simulink model "wwtp"  (R2022a)
settings: Solver=ode23t  StartTime=0.0  StopTime=inf  FixedStep=1E-4  MaxStep=100  RelTol=1e-4  EnableMultiTasking=on
InitFcn:
  | iniASU_UNIT
model workspace (MAT data in the model file):
  Port = 10001
  Port2 = 50001
  RemoteIP = '0.0.0.0'
values from neighbouring files (symbols this model uses):
  Arrhenius = ones(1,15)    [iniASM1model.m]
  Esteq = zeros(NUMREACCIONESBIOL,NUMESTADOSMODASM1)    [iniASM1model.m]
undefined symbols (not defined in the file or in its folder): Cineticos20, Param_ASU_D, Param_ASU_N, Param_Settler_Fns, ParamsEsteq, VarManip_D, VarManip_N, VarManip_QRF, x0_D, x0_N
libraries: dspnetwork x7
settings Model: PacingRate=0.890000  Creator=iirizar  LastModifiedBy=operezdearriluzea
settings SolverCC: InitialStep=1E-22  MaxConsecutiveMinStep=auto  AlgebraicLoopSolver=TrustRegion  SolverResetMethod=Robust
settings DataIOCC: LimitDataPoints=on  MaxDataPoints=1  SaveFinalState=on  SaveFormat=Array  SignalLoggingSaveFormat=ModelDataLogs  SaveOutput=off  SaveState=on  SignalLogging=off  SaveTime=off  ReturnWorkspaceOutputs=off
settings OptimizationCC: ExpressionDepthLimit=2147483647  LifeSpan=inf
settings DebuggingCC: UnderspecifiedInitializationDetection=Classic  MergeDetectMultiDrivingBlocksExec=none  SolverPrmCheckMsg=warning  FcnCallInpInsideContextMsg=warning  UnconnectedInputMsg=warning  UnconnectedOutputMsg=warning  UnconnectedLineMsg=warning  StateNameClashWarn=warning  SFUnexpectedBacktrackingDiag=warning  SFNoUnconditionalDefaultTransitionDiag=warning  SFExecutionAtInitializationDiag=none  SFMachineParentedDataDiag=warning  ArithmeticOperatorsInVariantConditions=warning
settings HardwareCC: ProdBitPerPointer=32  ProdBitPerSizeT=32  ProdBitPerPtrDiffT=32  ProdLargestAtomicFloat=None  ProdIntDivRoundTo=Undefined  ProdEndianess=Unspecified  ProdWordSize=32  ProdHWDeviceType=32-bit Generic
settings ModelReferenceCC: PropagateSignalLabelsOutOfModel=off
settings SFSimCC: SimUseLocalCustomCode=off  CustomCodeUndefinedFunction=UseInterfaceOnly
settings RTWCC: RTWUseLocalCustomCode=off  DLArmComputeVersion=19.05
settings CodeAppCC: StateflowObjectComments=on
settings GRTTargetCC: TargetLangStandard=C89/C90 (ANSI)  CombineOutputUpdateFcns=off  GRTInterface=on
settings ConfigComp: CovMetricSettings=dw  CovSaveCumulativeToWorkspaceVar=on  CovSaveSingleToWorkspaceVar=on  CovExternalEMLEnable=off

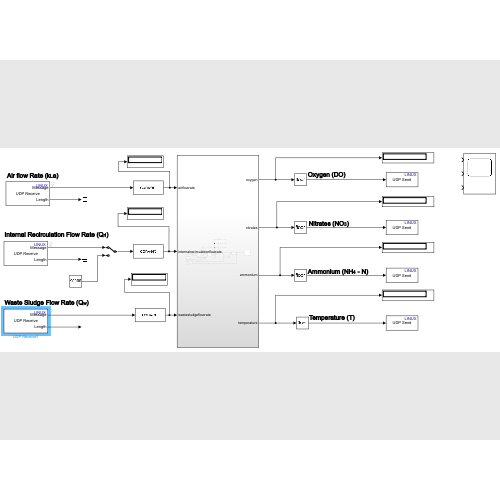
[thumbnail: Simulink's stored preview of the top-level diagram]
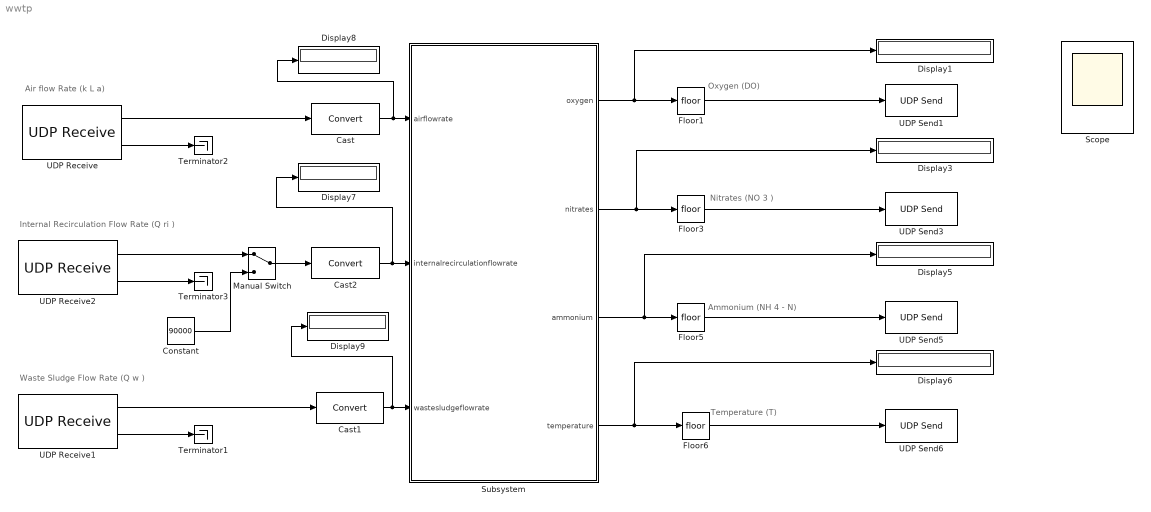
== system wwtp ==
  note: Air flow Rate (k L a)
  note: Waste Sludge Flow Rate (Q w )
  note: Internal Recirculation Flow Rate (Q ri )
  note: Oxygen (DO)
  note: Nitrates (NO 3 )
  note: Ammonium (NH 4 - N)
  note: Temperature (T)
  Cast : DataTypeConversion  OutMin=[0]  OutMax=[1000]  SaturateOnIntegerOverflow=off  RndMeth=Floor
  Cast1 : DataTypeConversion  OutMin=[0]  OutMax=[10000]  SaturateOnIntegerOverflow=off  RndMeth=Floor
  Cast2 : DataTypeConversion  OutMin=[0]  OutMax=[100000]  SaturateOnIntegerOverflow=off  RndMeth=Floor
  Constant : Constant  Value=90000
  Display{1,3,5..9} (7 alike) : Display
  Floor{1,3,5..6} (4 alike) : Rounding
  Manual Switch : ManualSwitch
  Scope : Scope  NumInputPorts=3
  Subsystem : Subsystem
  Terminator1 : Terminator
  Terminator2 : Terminator
  Terminator3 : Terminator
  UDP Receive : dspnetwork/UDP Receive  localURL='0.0.0.0'  localPort=50003  remoteURL='192.168.192.3'  remotePort=-1  recvBufferSize=2  dims=1  signalDatatype=uint16  isComplex=off  isVarSize=off  showBlockingTime=on  blockingTime=0  sampletime=0.1  blockPlatform=LINUX
  UDP Receive1 : dspnetwork/UDP Receive  localURL='0.0.0.0'  localPort=50002  remoteURL='192.168.192.3'  remotePort=-1  recvBufferSize=2  dims=1  signalDatatype=uint16  isComplex=off  isVarSize=off  showBlockingTime=on  blockingTime=0  sampletime=0.1  blockPlatform=LINUX
  UDP Receive2 : dspnetwork/UDP Receive  localURL='0.0.0.0'  localPort=50001  remoteURL='192.168.192.3'  remotePort=-1  recvBufferSize=2  dims=1  signalDatatype=uint16  isComplex=off  isVarSize=off  showBlockingTime=on  blockingTime=0  sampletime=0.1  blockPlatform=LINUX
  UDP Send1 : dspnetwork/UDP Send  remoteURL='192.168.192.2'  remotePort=10001  localURL='255.255.255.255'  localPortSource=Automatically determine  localPort=-1  sendBufferSize=8192*2  sampletime=-1  blockPlatform=LINUX  separateLengthPort=0
  UDP Send3 : dspnetwork/UDP Send  remoteURL='192.168.192.2'  remotePort=10002  localURL='255.255.255.255'  localPortSource=Automatically determine  localPort=-1  sendBufferSize=8192*2  sampletime=-1  blockPlatform=LINUX  separateLengthPort=0
  UDP Send5 : dspnetwork/UDP Send  remoteURL='192.168.192.2'  remotePort=10003  localURL='255.255.255.255'  localPortSource=Automatically determine  localPort=-1  sendBufferSize=8192*2  sampletime=-1  blockPlatform=LINUX  separateLengthPort=0
  UDP Send6 : dspnetwork/UDP Send  remoteURL='192.168.192.2'  remotePort=10004  localURL='255.255.255.255'  localPortSource=Automatically determine  localPort=-1  sendBufferSize=8192*2  sampletime=-1  blockPlatform=LINUX  separateLengthPort=0
  wires:
  UDP Receive1/2 -> Terminator1/1
  UDP Receive2/2 -> Terminator3/1
  UDP Receive/2 -> Terminator2/1
  UDP Receive/1 -> Cast/1
  UDP Receive1/1 -> Cast1/1
  Cast/1 -> Display8/1, Subsystem/1(airflowrate)
  Cast2/1 -> Subsystem/2(internalrecirculationflowrate), Display7/1
  Cast1/1 -> Display9/1, Subsystem/3(wastesludgeflowrate)
  Floor1/1 -> UDP Send1/1
  Subsystem/1(oxygen) -> Display1/1, Floor1/1
  Subsystem/2(nitrates) -> Floor3/1, Display3/1
  Floor3/1 -> UDP Send3/1
  Subsystem/3(ammonium) -> Display5/1, Floor5/1
  Floor5/1 -> UDP Send5/1
  Subsystem/4(temperature) -> Display6/1, Floor6/1
  Floor6/1 -> UDP Send6/1
  UDP Receive2/1 -> Manual Switch/1
  Constant/1 -> Manual Switch/2
  Manual Switch/1 -> Cast2/1

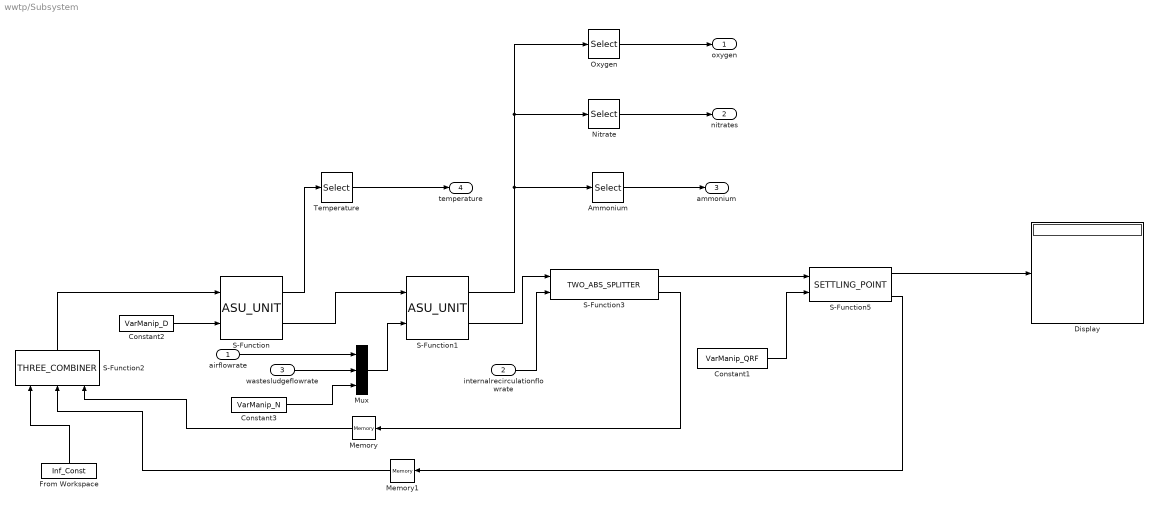
== system wwtp/Subsystem ==
  airflowrate : Inport
  internalrecirculationflowrate : Inport  Port=2
  wastesludgeflowrate : Inport  Port=3
  Ammonium : Selector  InputPortWidth=9  IndexOptions=Index vector (dialog)  Indices=[4]  OutputSizes=1
  Constant1 : Constant  Value=VarManip_QRF
  Constant2 : Constant  Value=VarManip_D
  Constant3 : Constant  Value=VarManip_N
  Display : Display
  From Workspace : FromWorkspace  VariableName=Inf_Const  Interpolate=off  OutputAfterFinalValue=Holding final value
  Memory : Memory  InheritSampleTime=on
  Memory1 : Memory  InheritSampleTime=on
  Mux : Mux  Inputs=3
  Nitrate : Selector  InputPortWidth=9  IndexOptions=Index vector (dialog)  Indices=[3]  OutputSizes=1
  Oxygen : Selector  InputPortWidth=9  IndexOptions=Index vector (dialog)  Indices=[5]  OutputSizes=1
  S-Function : S-Function  FunctionName=ASU_UNIT  Parameters=ParamsEsteq,Cineticos20,Arrhenius,Esteq,Param_ASU_D,x0_D  SFunctionDeploymentMode=off  EnableBusSupport=off
  S-Function1 : S-Function  FunctionName=ASU_UNIT  Parameters=ParamsEsteq,Cineticos20,Arrhenius,Esteq,Param_ASU_N,x0_N  SFunctionDeploymentMode=off  EnableBusSupport=off
  S-Function2 : S-Function  FunctionName=THREE_COMBINER  SFunctionDeploymentMode=off  EnableBusSupport=off
  S-Function3 : S-Function  FunctionName=TWO_ABS_SPLITTER  SFunctionDeploymentMode=off  EnableBusSupport=off
  S-Function5 : S-Function  FunctionName=SETTLING_POINT  Parameters=ParamsEsteq,Param_Settler_Fns  SFunctionDeploymentMode=off  EnableBusSupport=off
  Temperature : Selector  InputPortWidth=9  IndexOptions=Index vector (dialog)  Indices=[8]  OutputSizes=1
  oxygen : Outport
  nitrates : Outport  Port=2
  ammonium : Outport  Port=3
  temperature : Outport  Port=4
  wires:
  Constant2/1 -> S-Function/2
  Constant1/1 -> S-Function5/2
  airflowrate/1 -> Mux/1
  Mux/1 -> S-Function1/2
  Constant3/1 -> Mux/3
  S-Function/2 -> S-Function1/1
  Memory1/1 -> S-Function2/2
  S-Function2/1 -> S-Function/1
  Memory/1 -> S-Function2/3
  S-Function5/3 -> Memory1/1
  S-Function1/2 -> S-Function3/1
  S-Function3/2 -> Memory/1
  S-Function3/1 -> S-Function5/1
  From Workspace/1 -> S-Function2/1
  internalrecirculationflowrate/1 -> S-Function3/2
  wastesludgeflowrate/1 -> Mux/2
  Oxygen/1 -> oxygen/1
  Nitrate/1 -> nitrates/1
  Ammonium/1 -> ammonium/1
  S-Function/1 -> Temperature/1
  Temperature/1 -> temperature/1
  S-Function1/1 -> Oxygen/1, Nitrate/1, Ammonium/1
  S-Function5/1 -> Display/1
